simulink model "SimulinkV1"  (R2023a)
settings: Solver=VariableStepAuto  StartTime=0.0  StopTime=10  RelTol=1e-3
settings Model: Creator=noor6  LastModifiedBy=irfan
settings OptimizationCC: ReuseModelBlockBuffer=off

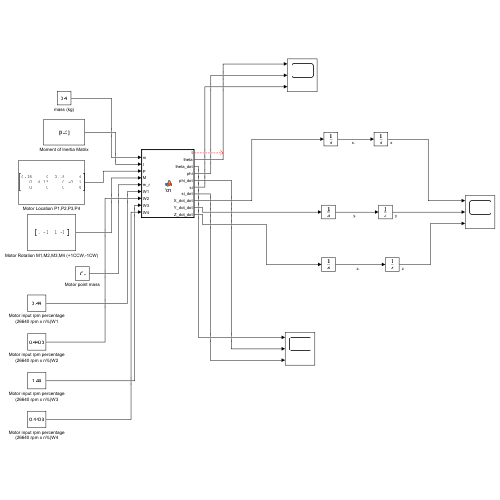
[thumbnail: Simulink's stored preview of the top-level diagram]
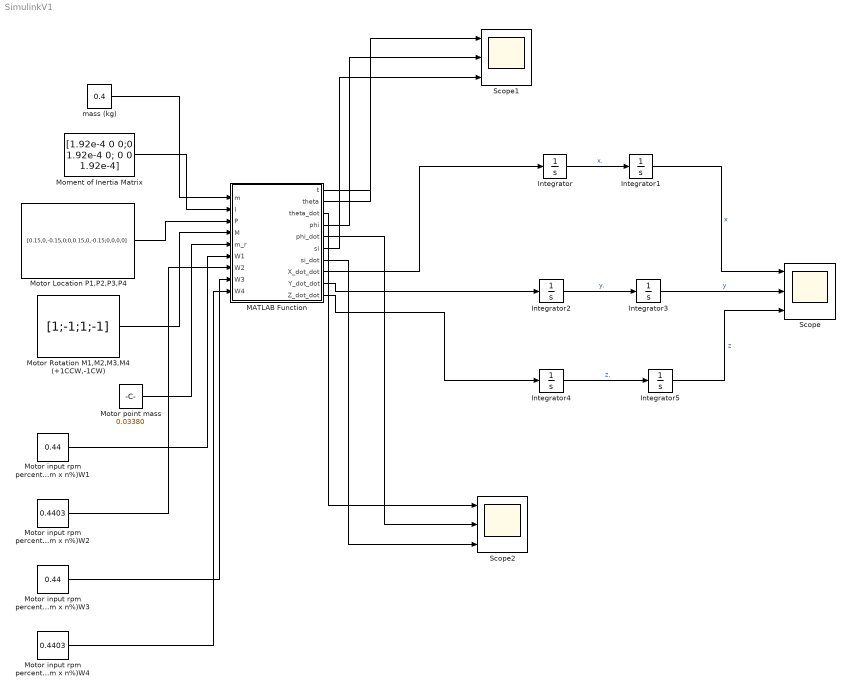
== system SimulinkV1 ==
  Integrator{,1..5} (6 alike) : Integrator
  MATLAB Function : MATLAB Function  TreatAsAtomicUnit=on
  Moment of Inertia Matrix : Constant  Value=[1.92e-4 0 0;0 1.92e-4 0; 0 0 1.92e-4]
  Motor Location P1,P2,P3,P4 : Constant  Value=[0.15,0,-0.15,0;0,0.15,0,-0.15;0,0,0,0]
  Motor Rotation M1,M2,M3,M4 (+1CCW,-1CW) : Constant  Value=[1;-1;1;-1]
  Motor input rpm percentage (26640 rpm x n%)W1 : Constant  Value=0.44
  Motor input rpm percentage (26640 rpm x n%)W2 : Constant  Value=0.4403
  Motor input rpm percentage (26640 rpm x n%)W3 : Constant  Value=0.44
  Motor input rpm percentage (26640 rpm x n%)W4 : Constant  Value=0.4403
  Motor point mass : Constant  Value=0.03380
  Scope : Scope  NumInputPorts=3
  Scope1 : Scope  NumInputPorts=3
  Scope2 : Scope  NumInputPorts=3
  mass (kg) : Constant  Value=0.4
  wires:
  Moment of Inertia Matrix/1 -> MATLAB Function/2(I)
  mass (kg)/1 -> MATLAB Function/1(m)
  Motor point mass/1 -> MATLAB Function/5(m_r)
  Motor Location P1,P2,P3,P4/1 -> MATLAB Function/3(P)
  Motor Rotation M1,M2,M3,M4 (+1CCW,-1CW)/1 -> MATLAB Function/4(M)
  MATLAB Function/2(theta) -> Scope1/1
  MATLAB Function/3(theta_dot) -> Scope2/1
  MATLAB Function/4(phi) -> Scope1/2
  MATLAB Function/5(phi_dot) -> Scope2/2
  MATLAB Function/7(si_dot) -> Scope2/3
  Integrator5/1 -> Scope/3  "z"
  Integrator1/1 -> Scope/1  "x"
  Integrator3/1 -> Scope/2  "y"
  Integrator4/1 -> Integrator5/1  "z."
  Integrator/1 -> Integrator1/1  "x."
  Integrator2/1 -> Integrator3/1  "y."
  MATLAB Function/6(si) -> Scope1/3
  MATLAB Function/8(X_dot_dot) -> Integrator/1
  MATLAB Function/9(Y_dot_dot) -> Integrator2/1
  MATLAB Function/10(Z_dot_dot) -> Integrator4/1
  MATLAB Function/1(t) -> ?
  Motor input rpm percentage (26640 rpm x n%)W1/1 -> MATLAB Function/6(W1)
  Motor input rpm percentage (26640 rpm x n%)W2/1 -> MATLAB Function/7(W2)
  Motor input rpm percentage (26640 rpm x n%)W3/1 -> MATLAB Function/8(W3)
  Motor input rpm percentage (26640 rpm x n%)W4/1 -> MATLAB Function/9(W4)

== matlab function SimulinkV1/MATLAB Function ==
  data: m input; t output; I input; P input; M input; m_r input; theta output; theta_dot output; phi output; phi_dot output; si output; si_dot output; X_dot_dot output; Y_dot_dot output; Z_dot_dot output; W1 input; W2 input; W3 input; W4 input
function [t,theta,theta_dot,phi,phi_dot,si,si_dot, X_dot_dot, Y_dot_dot, Z_dot_dot] = fcn(m,I,P,M,m_r,W1,W2,W3,W4)


coder.extrinsic('Anglecalc');


[J1,J2,size,accel]=Anglecalc(m,I,P,M,m_r,W1,W2,W3,W4);

% make the s variable 

s=11;
M=zeros(s,6);
M=J2;
N=zeros(s,3);
N=accel;

t=zeros(s,1);
t=J1;

theta=zeros(s,1);
theta_dot=zeros(s,1);
theta=M(:,1);
theta_dot=M(:,2);

phi=zeros(s,1);
phi_dot=zeros(s,1);
phi=M(:,3);
phi_dot=M(:,4);

si=zeros(s,1);
si_dot=zeros(s,1);
si=M(:,5);
si_dot=M(:,6);

X_dot_dot=zeros(s,1);
X_dot_dot=N(:,1);
Y_dot_dot=zeros(s,1);
Y_dot_dot=N(:,2);
Z_dot_dot=zeros(s,1);
Z_dot_dot=N(:,3);

end
